simulink model "BESS"  (R2024b)
settings: Solver=VariableStepAuto  StartTime=0  StopTime=4  FixedStep=1  MaxStep=1e-5  RelTol=1e-3
InitFcn:
  | t_stop = str2double(get_param('BESS', 'StopTime'));
undefined symbols (not defined in the file): Ion, Lithium
libraries: spsSeriesRLCBranchLib x6, spsVariableInductorLib x3, spsVariableResistorLib x3, spsBatteryLib x1, spsCurrentMeasurementLib x1, spsPWMGeneratorDCDCLib x1, spsPVArrayLib x1, spsPower3phInstantaneousLib x1, spsThreePhaseVIMeasurementLib x1, spsTwoQuadrantDCDCConverterLib x1, spsVoltageMeasurementLib x1, sps_lib x1
settings Model: Creator=mitphanase  LastModifiedBy=mitphanase
settings SolverCC: EnableFixedStepZeroCrossing=on

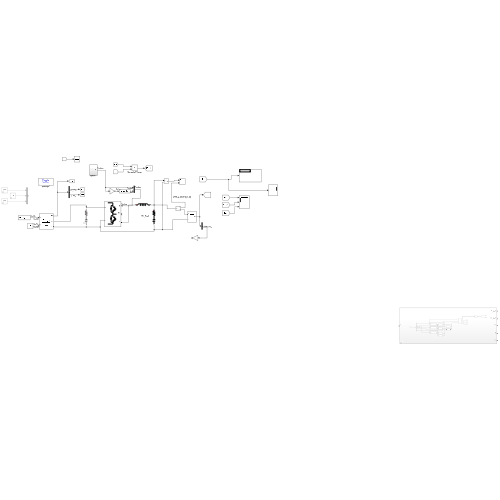
[thumbnail: Simulink's stored preview of the top-level diagram]
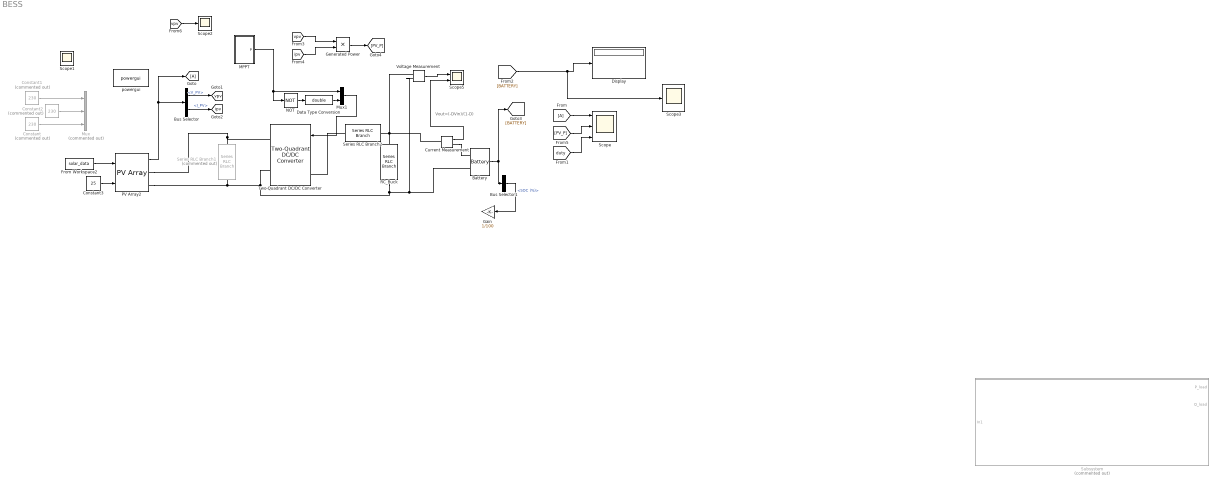
== system BESS ==
  note: Vout=(-DVin)/(1-D)
  Battery : spsBatteryLib/Battery  BatType=Lithium-Ion  NomV=400  NomQ=20  SOC=10  Batt_Tr=1  PresetModel=on  MaxQ=20  MinV=300  FullV=465.5949  Dis_rate=8.6957  R=0.2  Normal_OP=18.087  expZone="[432.1543     0.9826087]"
  Bus Selector : BusSelector  OutputSignals=V_PV,I_PV
  Bus Selector1 : BusSelector  OutputSignals=SOC (%)
  Constant : Constant  Commented=on  Value=230
  Constant1 : Constant  Commented=on  Value=230
  Constant2 : Constant  Commented=on  Value=230
  Constant3 : Constant  Value=25
  Current Measurement : spsCurrentMeasurementLib/Current Measurement  PhasorSimulation=off  OutputType=Complex  PSBequivalent=0
  Data Type Conversion : DataTypeConversion  OutDataTypeStr=double  SaturateOnIntegerOverflow=off  RndMeth=Floor
  Display : Display
  From : From
  From Workspace2 : FromWorkspace  VariableName=solar_data  OutDataTypeStr=double  SampleTime=1
  Gain : Gain  Gain=1/100
  Generated Power : Product
  Goto : Goto
  MPPT : Subsystem
  Mux : Mux  Commented=on  Inputs=3
  Mux1 : Mux  Inputs=2
  NOT : Logic  Operator=NOT  IconShape=distinctive  AllPortsSameDT=off  OutDataTypeStr=boolean
  PV Array2 : spsPVArrayLib/PV Array  Npar=4  Nser=7  PlotType=array @ 1000 W/m2 & specified temperatures  S_vec="[ 1000  500  100 ]"  Temp_C_vec="[ 45 25  ]"  ModuleName=SunPower SPR-415E-WHT-D  PlotWhenSelected=off  Pm=414.801  Ncell=128  Voc=85.3  Isc=6.09  Vm=72.9  Im=5.69  beta_Voc_pc=-0.229  alpha_Isc_pc=0.030706  beta_Voc=-0.19534  alpha_Isc=0.00187  IL=6.0978  I0=7.1698e-13  nI=0.87223  Rsh=419.7781  Rs=0.53711  RobustModel=off  RobustCellTemperature=313.3991  BAL=on  Tc=1e-6  Tfilter=5e-5
  RC_Buck : spsSeriesRLCBranchLib/Series RLC Branch  LConnTagsString=__new0  RConnTagsString=__new0  BranchType=RC  Resistance=1e-5  Inductance=1e-3  SetiL0=off  InitialCurrent=0  Capacitance=10e-6  Setx0=off  InitialVoltage=24  Measurements=Branch voltage and current
  Scope : Scope  NumInputPorts=3
  Scope2 : Scope
  Scope3 : Scope
  Scope5 : Scope  NumInputPorts=2
  Series RLC Branch1 : spsSeriesRLCBranchLib/Series RLC Branch  Commented=on  LConnTagsString=__new0  RConnTagsString=__new0  BranchType=RC  Resistance=1e-4  Inductance=1e-3  SetiL0=off  InitialCurrent=0  Capacitance=10e-6  Setx0=off  InitialVoltage=0  Measurements=Branch voltage
  Series RLC Branch2 : spsSeriesRLCBranchLib/Series RLC Branch  LConnTagsString=__new0  RConnTagsString=__new0  BranchType=L  Resistance=0.1  Inductance=10e-3  SetiL0=off  InitialCurrent=0  Capacitance=1e-6  Setx0=off  InitialVoltage=0  Measurements=Branch current
  Subsystem : Subsystem  Commented=on
  Two-Quadrant DC/DC Converter : spsTwoQuadrantDCDCConverterLib/Two-Quadrant DC//DC Converter  ModelType=Switching devices  Ron=1e-3  Rs=1e6  Cs=inf  Vforward=[0,0]  Ron_Diode=1e-3  Rs_Diode=1e6  Cs_Diode=inf  Vf_Diode=1e-3  Rs_CurrentSource=inf  Ron_ACsource=1e-3
  Voltage Measurement : spsVoltageMeasurementLib/Voltage Measurement  PhasorSimulation=off  OutputType=Complex  PSBequivalent=0
  powergui : sps_lib/powergui  Priority=1  SimulationMode=Discrete  SampleTime=1e-5  frequency=60  Iterations=50  frequencyindice=0  Pbase=100e6  ErrMax=1e-4  UnitsV=kV  UnitsW=MW  buscounter=0  FunctionMessages=off  echomessages=off  EnableUseOfTLC=off  CurrentSourceSwitches=off  DisableSnubberDevices=off  DisableRonSwitches=off  DisableVfSwitches=off  DisplayEquations=off  AutomaticDiscreteSolvers=off  SolverType=Tustin/Backward Euler (TBE)  Interpol=off  ExternalGateDelay=off  methode=off  Ts=100  x0status=blocks  SPID=on  SwTol=0  HookPort=off  NonlinearTolerance=1e-4  nMaxIteration=100  ContinueOnMaxIteration=off  RestoreLinks=warning  ResistiveCurrentMeasurement=off  Frange=[0:2:500]  Ylog=off  Xlog=on  ShowGrid=off  save=off  variable=ZData  structure=0  ZoomFFT=off  StartTime=0.0  cycles=1  DisplayStyle=1  fundamental=60  FreqAxis=off  MaxFrequency=1000  frequencyindicesteady=1  RmsSteady=1  display=off
  Scope1 : Scope
  tag scope: ipv=global, vpv=global
  wires:
  PV Array2/1 -> Goto/1, Bus Selector/1
  From/1 -> Scope/1
  Constant3/1 -> PV Array2/2
  Bus Selector/1 -> [vpv]  "<V_PV>"
  Bus Selector/2 -> [ipv]  "<I_PV>"
  Battery/1 -> Bus Selector1/1, [BATTERY]
  [BATTERY] -> Scope3/1, Display/1
  [vpv] -> Generated Power/1
  [ipv] -> Generated Power/2
  Generated Power/1 -> [PV_P]
  From Workspace2/1 -> PV Array2/1
  [PV_P] -> Scope/2
  MPPT/1(P) -> Mux1/1, NOT/1
  [vpv] -> Scope2/1
  Constant2/1 -> Mux/2
  Constant1/1 -> Mux/1
  Constant/1 -> Mux/3
  [duty] -> Scope/3
  Bus Selector1/1 -> Gain/1  "<SOC (%)>"
  Voltage Measurement/1 -> Scope5/1
  Current Measurement/1 -> Scope5/2
  Mux1/1 -> Two-Quadrant DC/DC Converter/1
  NOT/1 -> Data Type Conversion/1
  Data Type Conversion/1 -> Mux1/2
  connections:
  PV Array2/RConn1 -- Two-Quadrant DC/DC Converter/RConn1 -- Series RLC Branch1/LConn1
  Current Measurement/RConn1 -- Battery/LConn1
  Current Measurement/LConn1 -- Voltage Measurement/LConn1 -- RC_Buck/LConn1 -- Series RLC Branch2/RConn1
  PV Array2/RConn2 -- Two-Quadrant DC/DC Converter/RConn2 -- Voltage Measurement/LConn2 -- Battery/LConn2 -- RC_Buck/RConn1 -- Series RLC Branch1/RConn1
  Series RLC Branch2/LConn1 -- Two-Quadrant DC/DC Converter/LConn1

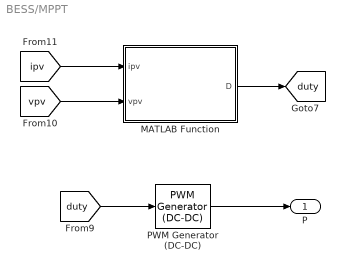
== system BESS/MPPT ==
  MATLAB Function : MATLAB Function  TreatAsAtomicUnit=on
  PWM Generator (DC-DC) : spsPWMGeneratorDCDCLib/PWM Generator (DC-DC)  Fsw=1000  Ts=0
  P : Outport
  tag scope: duty=global
  wires:
  [duty] -> PWM Generator (DC-DC)/1
  MATLAB Function/1(D) -> [duty]
  PWM Generator (DC-DC)/1 -> P/1
  [ipv] -> MATLAB Function/1(ipv)
  [vpv] -> MATLAB Function/2(vpv)

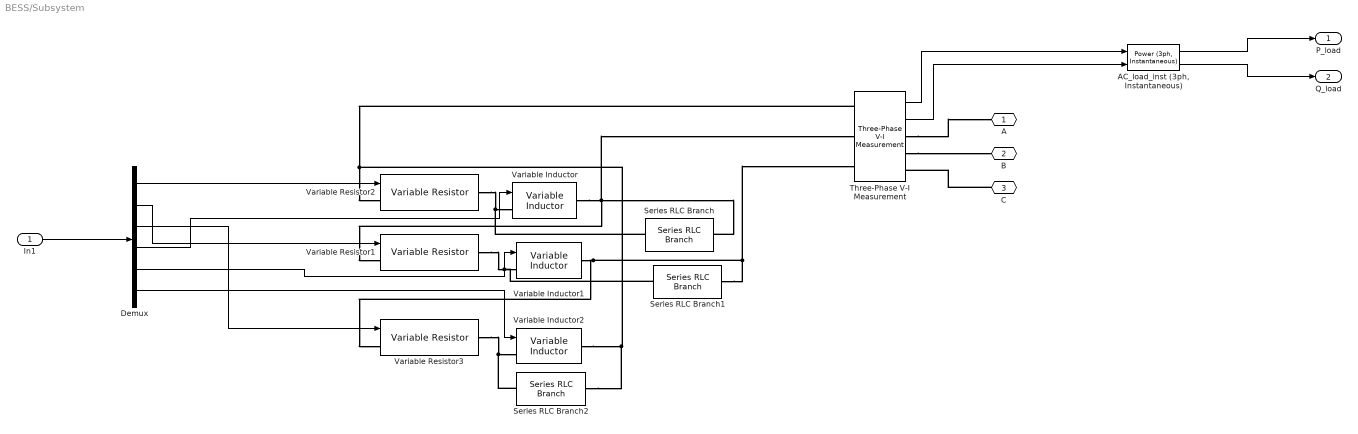
== system BESS/Subsystem ==
  In1 : Inport
  "AC_load_inst (3ph, Instantaneous)" : spsPower3phInstantaneousLib/Power (3ph, Instantaneous)
  Demux : Demux  Outputs=6
  Series RLC Branch : spsSeriesRLCBranchLib/Series RLC Branch  LConnTagsString=__new0  RConnTagsString=__new0  BranchType=R  Resistance=1e3  Inductance=0  SetiL0=off  InitialCurrent=0  Capacitance=0  Setx0=off  InitialVoltage=0  Measurements=None
  Series RLC Branch1 : spsSeriesRLCBranchLib/Series RLC Branch  LConnTagsString=__new0  RConnTagsString=__new0  BranchType=R  Resistance=1e3  Inductance=0  SetiL0=off  InitialCurrent=0  Capacitance=0  Setx0=off  InitialVoltage=0  Measurements=None
  Series RLC Branch2 : spsSeriesRLCBranchLib/Series RLC Branch  LConnTagsString=__new0  RConnTagsString=__new0  BranchType=R  Resistance=1e3  Inductance=0  SetiL0=off  InitialCurrent=0  Capacitance=0  Setx0=off  InitialVoltage=0  Measurements=None
  Three-Phase V-I Measurement : spsThreePhaseVIMeasurementLib/Three-Phase V-I Measurement  VoltageMeasurement=phase-to-phase  SetLabelV=off  LabelV=Vabc  Vpu=off  VpuLL=off  CurrentMeasurement=yes  SetLabelI=off  LabelI=Iabc  Ipu=off  Pbase=100e6  Vbase=500e3  OutputType=Complex  PhasorSimulation=off  PSBequivalent=0
  Variable Inductor : spsVariableInductorLib/Variable Inductor  methode=Backward Euler  Labsmin=1e-6  Initialize=off  iL0=0  L0=1e-3  Vl0=0
  Variable Inductor1 : spsVariableInductorLib/Variable Inductor  methode=Backward Euler  Labsmin=1e-6  Initialize=off  iL0=0  L0=1e-3  Vl0=0
  Variable Inductor2 : spsVariableInductorLib/Variable Inductor  methode=Backward Euler  Labsmin=1e-6  Initialize=off  iL0=0  L0=1e-3  Vl0=0
  Variable Resistor1 : spsVariableResistorLib/Variable Resistor  Rabsmin=1e-3
  Variable Resistor2 : spsVariableResistorLib/Variable Resistor  Rabsmin=1e-3
  Variable Resistor3 : spsVariableResistorLib/Variable Resistor  Rabsmin=1e-3
  "A " : PMIOPort  Side=Right
  " B" : PMIOPort  Port=2  Side=Right
  " C" : PMIOPort  Port=3  Side=Right
  P_load : Outport
  Q_load : Outport  Port=2
  wires:
  Demux/2 -> Variable Resistor1/1
  Demux/5 -> Variable Inductor1/1
  Demux/3 -> Variable Resistor3/1
  Demux/1 -> Variable Resistor2/1
  Demux/4 -> Variable Inductor/1
  Demux/6 -> Variable Inductor2/1
  In1/1 -> Demux/1
  Three-Phase V-I Measurement/1 -> "AC_load_inst (3ph, Instantaneous)"/1
  Three-Phase V-I Measurement/2 -> "AC_load_inst (3ph, Instantaneous)"/2
  "AC_load_inst (3ph, Instantaneous)"/1 -> P_load/1
  "AC_load_inst (3ph, Instantaneous)"/2 -> Q_load/1
  connections:
  Variable Resistor1/RConn1 -- Series RLC Branch1/LConn1 -- Variable Inductor1/LConn1
  Variable Inductor1/RConn1 -- Three-Phase V-I Measurement/LConn3 -- Series RLC Branch1/RConn1 -- Variable Resistor3/LConn1
  Variable Resistor3/RConn1 -- Series RLC Branch2/LConn1 -- Variable Inductor2/LConn1
  Three-Phase V-I Measurement/LConn1 -- Variable Resistor2/LConn1 -- Series RLC Branch2/RConn1 -- Variable Inductor2/RConn1
  Variable Resistor2/RConn1 -- Series RLC Branch/LConn1 -- Variable Inductor/LConn1
  Variable Inductor/RConn1 -- Three-Phase V-I Measurement/LConn2 -- Series RLC Branch/RConn1 -- Variable Resistor1/LConn1
  Three-Phase V-I Measurement/RConn1 -- "A "/RConn1
  Three-Phase V-I Measurement/RConn2 -- " B"/RConn1
  " C"/RConn1 -- Three-Phase V-I Measurement/RConn3

== matlab function BESS/MPPT/MATLAB Function ==
  data: ipv input; D output; vpv input
function D = pno_mppt(ipv, vpv)
        % P&O MPPT algorithm for PV system (optimized for buck converter)
        % Inputs: ipv - PV current (A), vpv - PV voltage (V)
        % Output: D - Duty cycle (0.1 to 0.9)

        persistent P_prev V_prev D_prev;
        if isempty(P_prev)
            P_prev = 0;
            V_prev = 0;
            D_prev = 0.5;
        end

        delta_D = 0.01;
        D_min = 0.1;
        D_max = 0.9;

        if isnan(ipv) || isnan(vpv) || ipv < 0 || vpv < 0
            D = D_prev;
            return;
        end

        P = ipv * vpv;
        delta_P = P - P_prev;
        delta_V = vpv - V_prev;

        if delta_P > 0
            if delta_V > 0
                D = D_prev + delta_D; % Increase voltage (increase D for buck)
            else
                D = D_prev - delta_D; % Decrease voltage (decrease D)
            end
        else
            if delta_V > 0
                D = D_prev - delta_D; % Decrease voltage (decrease D)
            else
                D = D_prev + delta_D; % Increase voltage (increase D)
            end
        end

        D = min(D_max, max(D_min, D));
        P_prev = P;
        V_prev = vpv;
        D_prev = D;
    end
